simulink model "Main_Sim_noActuatorBlock"  (R2018b)
settings: Solver=FixedStepAuto  StartTime=0.0  StopTime=12000  FixedStep=simParams.sample_time_s  RelTol=1e-3  EnableMultiTasking=on
undefined symbols (not defined in the file): fswParams, simParams
libraries: actuators_lib x1, CDH_command_lib x1, Environment_lib x1, FSW_Lib x1, Sensors_Lib x1, satelliteDynamics_lib x1
settings Model: Creator=devantormey  LastModifiedBy=colem
settings OptimizationCC: LifeSpan=inf
settings DebuggingCC: SFUnexpectedBacktrackingDiag=warning  SFNoUnconditionalDefaultTransitionDiag=warning
settings SFSimCC: SimUseLocalCustomCode=off
settings RTWCC: RTWUseLocalCustomCode=off
settings CodeAppCC: StateflowObjectComments=on
settings GRTTargetCC: TargetLangStandard=C89/C90 (ANSI)  GeneratePreprocessorConditionals=Disable all
settings ConfigComp: CovMetricSettings=dw  CovHtmlReporting=on  CovSaveCumulativeToWorkspaceVar=on  CovSaveSingleToWorkspaceVar=on  CovExternalEMLEnable=off

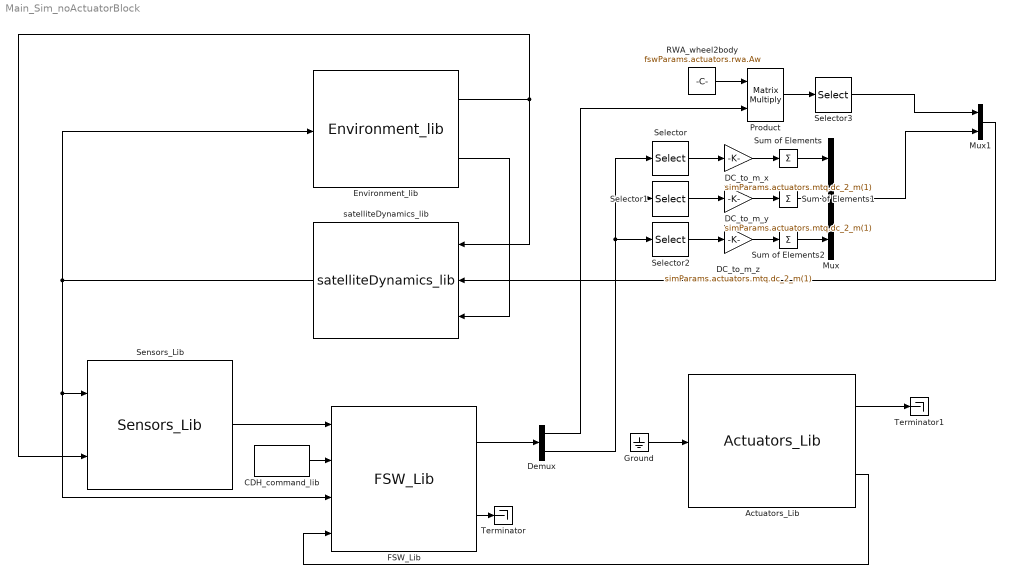
== system Main_Sim_noActuatorBlock ==
  Actuators_Lib : actuators_lib/Actuators_Lib  SystemSampleTime=-1
  CDH_command_lib : CDH_command_lib/CDH_command_lib  SystemSampleTime=-1
  DC_to_m_x : Gain  Gain=simParams.actuators.mtq.dc_2_m(1)
  DC_to_m_y : Gain  Gain=simParams.actuators.mtq.dc_2_m(1)
  DC_to_m_z : Gain  Gain=simParams.actuators.mtq.dc_2_m(1)
  Demux : Demux  Outputs=[4 5]
  Environment_lib : Environment_lib/Environment_lib  SystemSampleTime=-1
  FSW_Lib : FSW_Lib/FSW_Lib  SystemSampleTime=-1
  Ground : Ground
  Mux : Mux  Inputs=3
  Mux1 : Mux  Inputs=[3 3]
  Product : Product  Multiplication=Matrix(*)
  RWA_wheel2body : Constant  Value=fswParams.actuators.rwa.Aw
  Selector : Selector  InputPortWidth=sum(simParams.actuators.mtq.n_coils)  IndexOptions=Index vector (dialog)  Indices=simParams.actuators.mtq.id_x  OutputSizes=1
  Selector1 : Selector  InputPortWidth=sum(simParams.actuators.mtq.n_coils)  IndexOptions=Index vector (dialog)  Indices=simParams.actuators.mtq.id_y  OutputSizes=1
  Selector2 : Selector  InputPortWidth=sum(simParams.actuators.mtq.n_coils)  IndexOptions=Index vector (dialog)  Indices=simParams.actuators.mtq.id_z  OutputSizes=1
  Selector3 : Selector  InputPortWidth=4  IndexOptions=Index vector (dialog)  Indices=[1 2 3]  OutputSizes=1
  Sensors_Lib : Sensors_Lib/Sensors_Lib  SystemSampleTime=-1
      link override Goto3: GotoTag=B_eci_T
  Sum of Elements : Sum  Inputs=+
  Sum of Elements1 : Sum  Inputs=+
  Sum of Elements2 : Sum  Inputs=+
  Terminator : Terminator
  Terminator1 : Terminator
  satelliteDynamics_lib : satelliteDynamics_lib/satelliteDynamics_lib  SystemSampleTime=-1
  wires:
  FSW_Lib/1 -> Demux/1
  Sensors_Lib/1 -> FSW_Lib/1
  satelliteDynamics_lib/1 -> Environment_lib/1, FSW_Lib/3, Sensors_Lib/1
  Environment_lib/1 -> Sensors_Lib/2, satelliteDynamics_lib/1
  FSW_Lib/2 -> Terminator/1
  Actuators_Lib/2 -> FSW_Lib/4
  CDH_command_lib/1 -> FSW_Lib/2
  Actuators_Lib/1 -> Terminator1/1
  Environment_lib/2 -> satelliteDynamics_lib/3
  Ground/1 -> Actuators_Lib/1
  Demux/2 -> Selector1/1, Selector/1, Selector2/1
  Sum of Elements/1 -> Mux/1
  DC_to_m_x/1 -> Sum of Elements/1
  DC_to_m_z/1 -> Sum of Elements2/1
  Sum of Elements1/1 -> Mux/2
  Selector1/1 -> DC_to_m_y/1
  Sum of Elements2/1 -> Mux/3
  Mux/1 -> Mux1/2
  Selector2/1 -> DC_to_m_z/1
  DC_to_m_y/1 -> Sum of Elements1/1
  Selector/1 -> DC_to_m_x/1
  RWA_wheel2body/1 -> Product/1
  Selector3/1 -> Mux1/1
  Demux/1 -> Product/2
  Product/1 -> Selector3/1
  Mux1/1 -> satelliteDynamics_lib/2
